simulink model "gen_2_Neel"  (R2017a)
settings: Solver=VariableStepAuto  StartTime=0.0  StopTime=100  MaxStep=1e-4  RelTol=1e-3
libraries: powerlib x33, simrfV2util1 x6, simulink x6, simrfV2_lib x6, powerlib_meascontrol x4
settings Model: SimulationMode=accelerator  Creator=khsva  LastModifiedBy=Purboday Ghosh
settings SolverCC: ZeroCrossAlgorithm=Adaptive
settings OptimizationCC: EfficientMapNaN2IntZero=off
settings HardwareCC: TargetBitPerPointer=64  TargetBitPerSizeT=64  TargetBitPerPtrDiffT=64  TargetLongLongMode=on  TargetIntDivRoundTo=Zero  TargetEndianess=LittleEndian  TargetWordSize=64  TargetHWDeviceType=MATLAB Host  ProdEqTarget=off
settings CodeAppCC: MaxIdLength=128
settings GRTTargetCC: TargetLangStandard=C89/C90 (ANSI)  CombineOutputUpdateFcns=off  GRTInterface=on

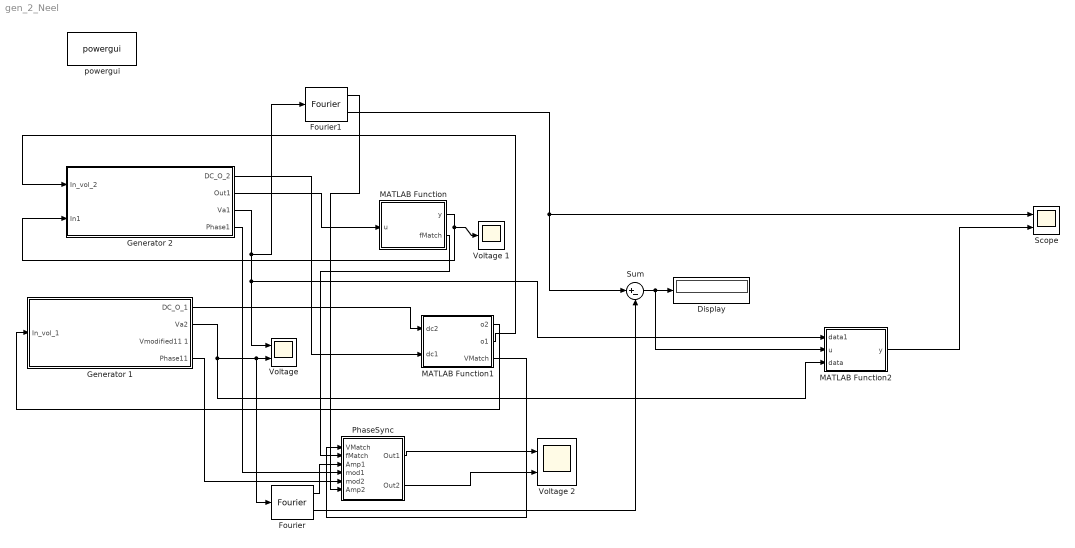
== system gen_2_Neel ==
  Display : Display
  Fourier : powerlib_meascontrol/Measurements/Fourier  Freq=60  n=1  InInit=[0, 0]  Ts=0
      settings: SourceProductName=Simscape Power Systems
  Fourier1 : powerlib_meascontrol/Measurements/Fourier  Freq=60  n=1  InInit=[0, 0]  Ts=0
      settings: SourceProductName=Simscape Power Systems
  "Generator 1 " : Subsystem
  Generator 2 : Subsystem
  MATLAB Function : MATLAB Function  TreatAsAtomicUnit=on
  MATLAB Function1 : MATLAB Function  TreatAsAtomicUnit=on
  MATLAB Function2 : MATLAB Function  TreatAsAtomicUnit=on
  PhaseSync : Subsystem
  Scope : Scope  NumInputPorts=2
  Sum : Sum  Inputs=|+-
  "Voltage " : Scope  NumInputPorts=2
  Voltage 1 : Scope
  Voltage 2 : Scope  NumInputPorts=2
  powergui : powerlib/powergui  Priority=1  SimulationMode=Continuous  SampleTime=50e-6  frequency=60  Iterations=50  frequencyindice=60  Pbase=100e6  ErrMax=1e-4  UnitsV=kV  UnitsW=MW  buscounter=0  FunctionMessages=off  echomessages=off  EnableUseOfTLC=off  CurrentSourceSwitches=off  DisableSnubberDevices=off  DisableRonSwitches=off  DisableVfSwitches=off  DisplayEquations=off  SolverType=Tustin/Backward Euler (TBE)  Interpol=off  ExternalGateDelay=off  methode=off  Ts=100  x0status=blocks  SPID=on  SwTol=0  HookPort=off  RestoreLinks=warning  ResistiveCurrentMeasurement=off  Frange=[0:2:500]  Ylog=off  Xlog=on  ShowGrid=off  save=off  variable=ZData  structure=0  ZoomFFT=off  StartTime=0.0  cycles=1  DisplayStyle=1  fundamental=60  FreqAxis=off  MaxFrequency=1000  frequencyindicesteady=1  RmsSteady=1  display=off
  wires:
  "Generator 1 "/1("DC_O_1 ") -> MATLAB Function1/1(dc2)
  Generator 2/1(DC_O_2) -> MATLAB Function1/2(dc1)
  MATLAB Function1/1(o2) -> "Generator 1 "/1("In_vol_1 ")
  MATLAB Function1/2(o1) -> Generator 2/1("In_vol_2 ")
  MATLAB Function/1(y) -> Voltage 1/1, Generator 2/2(In1)
  Generator 2/2(Out1) -> MATLAB Function/1(u)
  Generator 2/3(Va1) -> Fourier1/1, MATLAB Function2/1(data1), "Voltage "/1
  "Generator 1 "/2("Va2 ") -> MATLAB Function2/3(data), Fourier/1, "Voltage "/2
  Sum/1 -> MATLAB Function2/2(u), Display/1
  Fourier/2 -> Sum/2
  Fourier1/2 -> Sum/1, Scope/1
  MATLAB Function2/1(y) -> Scope/2
  "Generator 1 "/4(Phase11) -> PhaseSync/5(mod2)
  Generator 2/4(Phase1) -> PhaseSync/4(mod1)
  PhaseSync/1(Out1) -> Voltage 2/1
  PhaseSync/2(Out2) -> Voltage 2/2
  Fourier1/1 -> PhaseSync/6(Amp2)
  Fourier/1 -> PhaseSync/3(Amp1)
  MATLAB Function/2(fMatch) -> PhaseSync/2(fMatch)
  MATLAB Function1/3(VMatch) -> PhaseSync/1(VMatch)

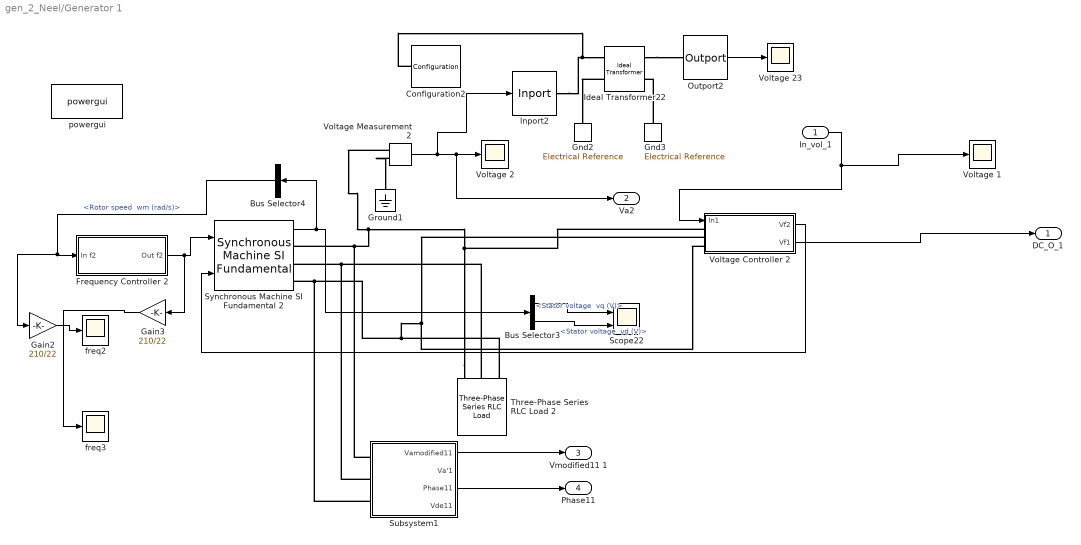
== system gen_2_Neel/Generator 1  ==
  "In_vol_1 " : Inport
  Bus Selector3 : BusSelector  OutputSignals="dq0 components.Stator voltage  vq (V),dq0 components.Stator voltage  vd (V)"
  Bus Selector4 : BusSelector  OutputSignals="Mechanical.Rotor speed  wm (rad/s)"
  Configuration2 : simrfV2util1/Configuration  AutoFreq=on  Tones=[0] Hz  Harmonics=[1]  NormalizeCarrierPower=on  SolverType=Auto  UseCCode=on  StepSize=1e-4 s  AddNoise=on  defaultRNG=on  Seed=0  Temperature=290.0 K  SolverDelFlag=0  AbsTol=1e-6  RelTol=1e-3  MaxIter=10  ErrorEstimationType=2-norm over all variables
      settings: SourceProductName=SimRF  SourceProductBaseCode=RB
  Frequency Controller 2 : Subsystem
  Gain2 : Gain  Gain=210/22
  Gain3 : Gain  Gain=210/22
  Gnd2 : simrfV2_lib/Elements/Electrical Reference
  Gnd3 : simrfV2_lib/Elements/Electrical Reference
  Ground1 : powerlib/Elements/Ground  LConnTagsString=a
  Ideal Transformer22 : simrfV2_lib/Elements/Ideal Transformer  n=10
  Inport2 : simrfV2util1/Inport  SimulinkInputSignalType=Ideal voltage  CarrierFreq=0 Hz  ZS=0  InternalGrounding=on
      settings: SourceProductName=SimRF  SourceProductBaseCode=RB
  Outport2 : simrfV2util1/Outport  SensorType=Ideal voltage  OutputFormat=Complex Baseband  CarrierFreq=0 Hz  ZL=Inf  InternalGrounding=on  StepSize=1e-6 s  AutoStep=on
      settings: SourceProductName=SimRF  SourceProductBaseCode=RB
  Scope22 : Scope  NumInputPorts=2
  Subsystem1 : Subsystem
  Synchronous Machine SI Fundamental 2 : powerlib/Machines/Synchronous Machine SI Fundamental  PresetModel=No  MechanicalLoad=Speed w  ShowDetailedParameters=on  RotorType=Salient-pole  Units=SI fundamental parameters  MeasurementBus=off  NominalParameters="[ 200E3  110   60   70 ]"  Stator="[ 200  3.0892  3.2164  9.7153 ]"  Field="[ 200  30.712 ]"  Dampers2=[ 0.0664, 1.387e-3, 0.0292, 6.896e-4, 7.907e-3, 2.477e-3]  Dampers1="[ 1.1900E-02  4.9076E-04  2.0081E-02  1.0365E-03 ]"  Mechanical=[ 3.895e6 0 20 ]  PolePairs=10  InitialConditions="[ 0  0  0  0  0  0  0  0  0 ]"  SetSaturation=off  Saturation=[695.64,774.7,917.5,1001.6,1082.2,1175.9,1293.6,1430.2,1583.7;9660,10623,12243,13063,13757,14437,15180,15890,16567]  DisplayVfd=off  LoadFlowParameters=[1,0,0,0,0]  TsPowergui=0  TsBlock=-1  IterativeModel=Trapezoidal non iterative  IterativeDiscreteModel=Trapezoidal non iterative  BusType=PV  Pref=0  Qref=0  Qmin=-inf  Qmax=inf  PLF=0  QLF=0
      settings: SourceProductName=Simscape Power Systems  SourceProductBaseCode=PS
  Three-Phase Series RLC Load 2 : powerlib/Elements/Three-Phase Series RLC Load  LConnTagsString=A|B|C  Configuration=Y (grounded)  NominalVoltage=100  Vabc=[1e3 1e3 1e3]  Vabcp=[1e3 1e3 1e3]  NominalFrequency=60  UnbalancedPower=off  ActivePower=2500  InductivePower=0  CapacitivePower=0  Pabc=[10e3 9e3 11e3]  QLabc=[100 90 110]  QCabc=[100 90 110]  Pabcp=[10e3 9e3 11e3]  QLabcp=[100 90 110]  QCabcp=[100 90 110]  Measurements=None  LoadType=constant Z
  Voltage 1 : Scope
  Voltage 2 : Scope
  Voltage 23 : Scope
  Voltage Controller 2 : Subsystem
  Voltage Measurement2 : powerlib/Measurements/Voltage Measurement  PhasorSimulation=off  OutputType=Complex  PSBequivalent=0
  freq2 : Scope
  freq3 : Scope
  powergui : powerlib/powergui  Priority=1  SimulationMode=Continuous  SampleTime=50e-6  frequency=60  Iterations=50  frequencyindice=60  Pbase=100e6  ErrMax=1e-4  UnitsV=kV  UnitsW=MW  buscounter=0  FunctionMessages=off  echomessages=off  EnableUseOfTLC=off  CurrentSourceSwitches=off  DisableSnubberDevices=off  DisableRonSwitches=off  DisableVfSwitches=off  DisplayEquations=off  SolverType=Tustin/Backward Euler (TBE)  Interpol=off  ExternalGateDelay=off  methode=off  Ts=100  x0status=blocks  SPID=on  SwTol=0  HookPort=off  RestoreLinks=warning  ResistiveCurrentMeasurement=off  Frange=[0:2:500]  Ylog=off  Xlog=on  ShowGrid=off  save=off  variable=ZData  structure=0  ZoomFFT=off  StartTime=0.0  cycles=1  DisplayStyle=1  fundamental=60  FreqAxis=off  MaxFrequency=1000  frequencyindicesteady=1  RmsSteady=1  display=off
  "DC_O_1 " : Outport
  "Va2 " : Outport  Port=2
  Vmodified11 1 : Outport  Port=3
  Phase11 : Outport  Port=4
  wires:
  Frequency Controller 2/1(Out f2) -> Gain3/1, Synchronous Machine SI Fundamental 2/1
  Bus Selector3/1 -> Scope22/1  "<Stator voltage  vq (V)>"
  Gain2/1 -> freq2/1
  Synchronous Machine SI Fundamental 2/1 -> Bus Selector4/1, Bus Selector3/1
  Outport2/1 -> Voltage 23/1
  Bus Selector4/1 -> Frequency Controller 2/1(In f2), Gain2/1  "<Rotor speed  wm (rad/s)>"
  Gain3/1 -> freq3/1
  Voltage Measurement2/1 -> Inport2/1, "Va2 "/1, Voltage 2/1
  Voltage Controller 2/1(Vf2) -> Synchronous Machine SI Fundamental 2/2
  Bus Selector3/2 -> Scope22/2  "<Stator voltage  vd (V)>"
  Voltage Controller 2/2(Vf1) -> "DC_O_1 "/1
  "In_vol_1 "/1 -> Voltage 1/1, Voltage Controller 2/1(In1)
  Subsystem1/1(Vamodified11) -> Vmodified11 1/1
  Subsystem1/3(Phase11) -> Phase11/1
  connections:
  Voltage Controller 2/LConn3 -- Voltage Controller 2/LConn2 -- Three-Phase Series RLC Load 2/LConn3 -- Subsystem1/LConn3 -- Synchronous Machine SI Fundamental 2/RConn3
  Voltage Measurement2/LConn2 -- Ground1/LConn1
  Gnd3/LConn1 -- Ideal Transformer22/RConn2
  Inport2/RConn1 -- Configuration2/LConn1 -- Ideal Transformer22/LConn1
  Three-Phase Series RLC Load 2/LConn2 -- Subsystem1/LConn2 -- Synchronous Machine SI Fundamental 2/RConn2
  Ideal Transformer22/RConn1 -- Outport2/LConn1
  Three-Phase Series RLC Load 2/LConn1 -- Voltage Controller 2/LConn1 -- Subsystem1/LConn1 -- Synchronous Machine SI Fundamental 2/RConn1 -- Voltage Measurement2/LConn1
  Ideal Transformer22/LConn2 -- Gnd2/LConn1

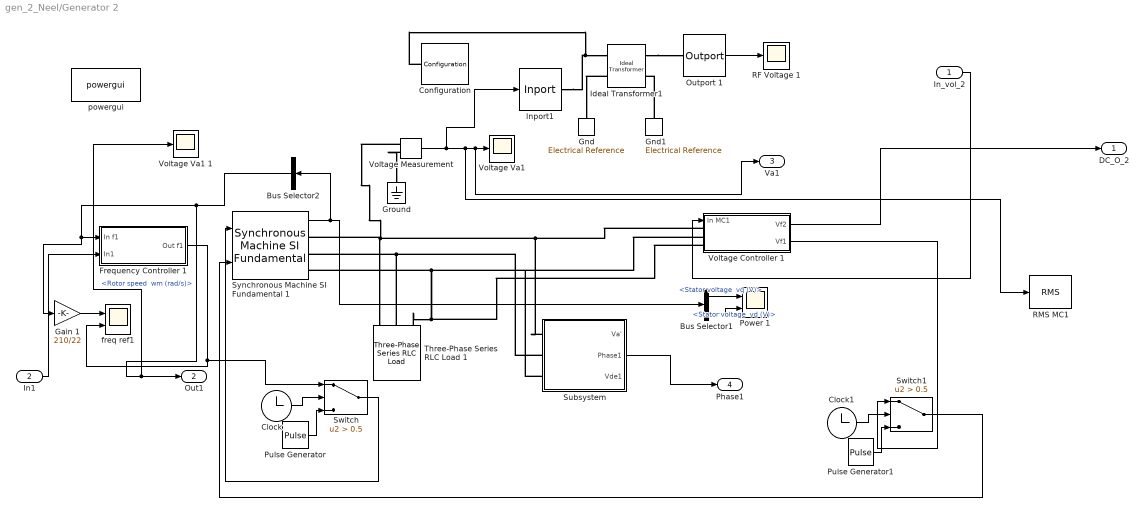
== system gen_2_Neel/Generator 2 ==
  "In_vol_2 " : Inport
  In1 : Inport  Port=2
  Bus Selector1 : BusSelector  OutputSignals="dq0 components.Stator voltage  vq (V),dq0 components.Stator voltage  vd (V)"
  Bus Selector2 : BusSelector  OutputSignals="Mechanical.Rotor speed  wm (rad/s)"
  Clock : Clock
  Clock1 : Clock
  Configuration : simrfV2util1/Configuration  AutoFreq=on  Tones=[0] Hz  Harmonics=[1]  NormalizeCarrierPower=on  SolverType=Auto  UseCCode=on  StepSize=1e-4 s  AddNoise=on  defaultRNG=on  Seed=0  Temperature=290.0 K  SolverDelFlag=0  AbsTol=1e-6  RelTol=1e-3  MaxIter=10  ErrorEstimationType=2-norm over all variables
      settings: SourceProductName=SimRF  SourceProductBaseCode=RB
  Frequency Controller 1 : Subsystem
  Gain 1 : Gain  Gain=210/22
  Gnd : simrfV2_lib/Elements/Electrical Reference
  Gnd1 : simrfV2_lib/Elements/Electrical Reference
  Ground : powerlib/Elements/Ground  LConnTagsString=a
  Ideal Transformer1 : simrfV2_lib/Elements/Ideal Transformer  n=10
  Inport1 : simrfV2util1/Inport  SimulinkInputSignalType=Ideal voltage  CarrierFreq=0 Hz  ZS=0  InternalGrounding=on
      settings: SourceProductName=SimRF  SourceProductBaseCode=RB
  Outport 1 : simrfV2util1/Outport  SensorType=Ideal voltage  OutputFormat=Complex Baseband  CarrierFreq=0 Hz  ZL=Inf  InternalGrounding=on  StepSize=1e-6 s  AutoStep=on
      settings: SourceProductName=SimRF  SourceProductBaseCode=RB
  Power 1 : Scope  NumInputPorts=2
  Pulse Generator : DiscretePulseGenerator  PulseType=Time based  Amplitude=0  Period=5  PulseWidth=99.99  PhaseDelay=0.5
  Pulse Generator1 : DiscretePulseGenerator  PulseType=Time based  Amplitude=0  Period=5  PulseWidth=99.99  PhaseDelay=0.5
  RF Voltage 1 : Scope
  RMS MC1 : powerlib_meascontrol/Measurements/RMS  TrueRMS=on  Freq=60  RMSInit=120  Ts=0
  Subsystem : Subsystem
  Switch : Switch  Criteria=u2 > Threshold  Threshold=0.5
  Switch1 : Switch  Criteria=u2 > Threshold  Threshold=0.5
  Synchronous Machine SI Fundamental 1 : powerlib/Machines/Synchronous Machine SI Fundamental  PresetModel=No  MechanicalLoad=Speed w  ShowDetailedParameters=on  RotorType=Salient-pole  Units=SI fundamental parameters  MeasurementBus=off  NominalParameters="[ 200E3  110   60   70 ]"  Stator="[ 200  3.0892  3.2164  9.7153 ]"  Field="[ 200  30.712 ]"  Dampers2=[ 0.0664, 1.387e-3, 0.0292, 6.896e-4, 7.907e-3, 2.477e-3]  Dampers1="[ 1.1900E-02  4.9076E-04  2.0081E-02  1.0365E-03 ]"  Mechanical=[ 3.895e6 0 20 ]  PolePairs=10  InitialConditions="[ 0  0  0  0  0  0  0  0  0 ]"  SetSaturation=off  Saturation=[695.64,774.7,917.5,1001.6,1082.2,1175.9,1293.6,1430.2,1583.7;9660,10623,12243,13063,13757,14437,15180,15890,16567]  DisplayVfd=off  LoadFlowParameters=[1,0,0,0,0]  TsPowergui=0  TsBlock=-1  IterativeModel=Trapezoidal non iterative  IterativeDiscreteModel=Trapezoidal non iterative  BusType=PV  Pref=0  Qref=0  Qmin=-inf  Qmax=inf  PLF=0  QLF=0
      settings: SourceProductName=Simscape Power Systems  SourceProductBaseCode=PS
  Three-Phase Series RLC Load 1 : powerlib/Elements/Three-Phase Series RLC Load  LConnTagsString=A|B|C  Configuration=Y (grounded)  NominalVoltage=100  Vabc=[1e3 1e3 1e3]  Vabcp=[1e3 1e3 1e3]  NominalFrequency=60  UnbalancedPower=off  ActivePower=1000  InductivePower=0  CapacitivePower=0  Pabc=[10e3 9e3 11e3]  QLabc=[100 90 110]  QCabc=[100 90 110]  Pabcp=[10e3 9e3 11e3]  QLabcp=[100 90 110]  QCabcp=[100 90 110]  Measurements=None  LoadType=constant Z
  Voltage Controller 1 : Subsystem
  Voltage Measurement : powerlib/Measurements/Voltage Measurement  PhasorSimulation=off  OutputType=Complex  PSBequivalent=0
  "Voltage Va1 " : Scope
  Voltage Va1 1 : Scope
  "freq ref1 " : Scope  NumInputPorts=2
  powergui : powerlib/powergui  Priority=1  SimulationMode=Continuous  SampleTime=50e-6  frequency=60  Iterations=50  frequencyindice=60  Pbase=100e6  ErrMax=1e-4  UnitsV=kV  UnitsW=MW  buscounter=0  FunctionMessages=off  echomessages=off  EnableUseOfTLC=off  CurrentSourceSwitches=off  DisableSnubberDevices=off  DisableRonSwitches=off  DisableVfSwitches=off  DisplayEquations=off  SolverType=Tustin/Backward Euler (TBE)  Interpol=off  ExternalGateDelay=off  methode=off  Ts=100  x0status=blocks  SPID=on  SwTol=0  HookPort=off  RestoreLinks=warning  ResistiveCurrentMeasurement=off  Frange=[0:2:500]  Ylog=off  Xlog=on  ShowGrid=off  save=off  variable=ZData  structure=0  ZoomFFT=off  StartTime=0.0  cycles=1  DisplayStyle=1  fundamental=60  FreqAxis=off  MaxFrequency=1000  frequencyindicesteady=1  RmsSteady=1  display=off
  DC_O_2 : Outport
  Out1 : Outport  Port=2
  Va1 : Outport  Port=3
  Phase1 : Outport  Port=4
  wires:
  Outport 1/1 -> RF Voltage 1/1
  Synchronous Machine SI Fundamental 1/1 -> Bus Selector2/1, Bus Selector1/1
  Gain 1/1 -> "freq ref1 "/1
  Frequency Controller 1/1(Out f1) -> Switch/1, "freq ref1 "/2
  Bus Selector1/1 -> Power 1/1  "<Stator voltage  vq (V)>"
  Bus Selector1/2 -> Power 1/2  "<Stator voltage  vd (V)>"
  Bus Selector2/1 -> Voltage Va1 1/1, Out1/1, Gain 1/1, Frequency Controller 1/1(In f1)  "<Rotor speed  wm (rad/s)>"
  "In_vol_2 "/1 -> Voltage Controller 1/1(In MC1)
  Voltage Measurement/1 -> Inport1/1, RMS MC1/1, Va1/1, "Voltage Va1 "/1
  Voltage Controller 1/1(Vf2) -> DC_O_2/1
  In1/1 -> Frequency Controller 1/2(In1)
  Clock/1 -> Switch/2
  Switch/1 -> Synchronous Machine SI Fundamental 1/1
  Pulse Generator/1 -> Switch/3
  Pulse Generator1/1 -> Switch1/3
  Clock1/1 -> Switch1/2
  Switch1/1 -> Synchronous Machine SI Fundamental 1/2
  Voltage Controller 1/2(Vf1) -> Switch1/1
  Subsystem/2(Phase1) -> Phase1/1
  connections:
  Inport1/RConn1 -- Configuration/LConn1 -- Ideal Transformer1/LConn1
  Ideal Transformer1/RConn1 -- Outport 1/LConn1
  Ideal Transformer1/LConn2 -- Gnd/LConn1
  Gnd1/LConn1 -- Ideal Transformer1/RConn2
  Voltage Controller 1/LConn1 -- Subsystem/LConn1 -- Voltage Measurement/LConn1 -- Synchronous Machine SI Fundamental 1/RConn1 -- Three-Phase Series RLC Load 1/LConn1
  Voltage Measurement/LConn2 -- Ground/LConn1
  Three-Phase Series RLC Load 1/LConn3 -- Subsystem/LConn3 -- Voltage Controller 1/LConn2 -- Synchronous Machine SI Fundamental 1/RConn3 -- Voltage Controller 1/LConn3
  Three-Phase Series RLC Load 1/LConn2 -- Synchronous Machine SI Fundamental 1/RConn2 -- Subsystem/LConn2

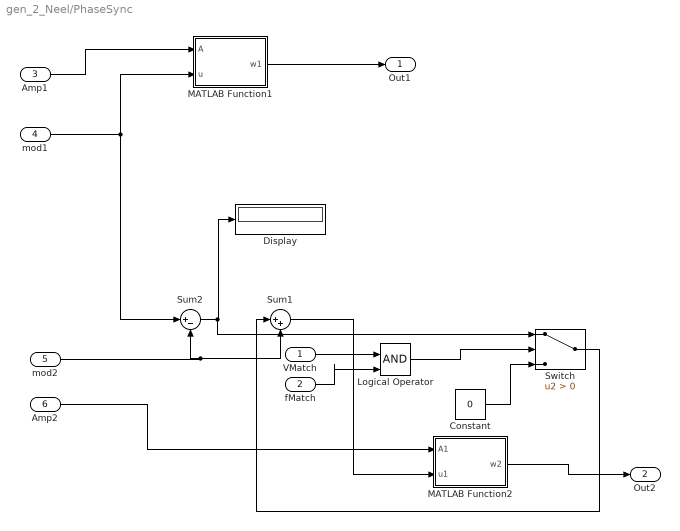
== system gen_2_Neel/PhaseSync ==
  VMatch : Inport
  fMatch : Inport  Port=2
  Amp1 : Inport  Port=3
  mod1 : Inport  Port=4
  mod2 : Inport  Port=5
  Amp2 : Inport  Port=6
  Constant : Constant  Value=0
  Display : Display
  Logical Operator : Logic  IconShape=distinctive  AllPortsSameDT=off  OutDataTypeStr=boolean
  MATLAB Function1 : MATLAB Function  TreatAsAtomicUnit=on
  MATLAB Function2 : MATLAB Function  TreatAsAtomicUnit=on
  Sum1 : Sum  Inputs=|++
  Sum2 : Sum  Inputs=|+-
  Switch : Switch  Criteria=u2 > Threshold
  Out1 : Outport
  Out2 : Outport  Port=2
  wires:
  Sum2/1 -> Switch/1, Display/1
  Sum1/1 -> MATLAB Function2/2(u1)
  MATLAB Function2/1(w2) -> Out2/1
  MATLAB Function1/1(w1) -> Out1/1
  Amp1/1 -> MATLAB Function1/1(A)
  Amp2/1 -> MATLAB Function2/1(A1)
  mod2/1 -> Sum1/2, Sum2/2
  Logical Operator/1 -> Switch/2
  Constant/1 -> Switch/3
  Switch/1 -> Sum1/1
  mod1/1 -> MATLAB Function1/2(u), Sum2/1
  fMatch/1 -> Logical Operator/2
  VMatch/1 -> Logical Operator/1

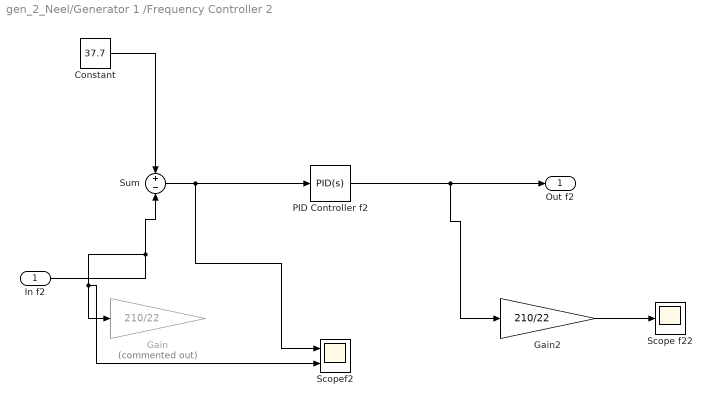
== system gen_2_Neel/Generator 1 /Frequency Controller 2 ==
  In f2 : Inport
  Constant : Constant  Value=37.7
  Gain : Gain  Commented=on  Gain=210/22
  Gain2 : Gain  Gain=210/22
  PID Controller f2 : simulink/Continuous/PID Controller  Controller=PID  TimeDomain=Continuous-time  SampleTime=-1  IntegratorMethod=Forward Euler  FilterMethod=Forward Euler  Form=Ideal  UseFilter=on  ControllerParametersSource=internal  P=9.99999998333334e-05  I=6309.57342377002  D=0  N=100  InitialConditionSource=internal  InitialConditionForIntegrator=0  InitialConditionForFilter=0  ExternalReset=none  LimitOutput=off  UpperSaturationLimit=inf  LowerSaturationLimit=-inf  LinearizeAsGain=on  AntiWindupMode=none  Kb=1  TrackingMode=off  Kt=1  PParamMin=[]  PParamMax=[]  IParamMin=[]  IParamMax=[]  DParamMin=[]  DParamMax=[]  NParamMin=[]  NParamMax=[]  KbParamMin=[]  KbParamMax=[]  KtParamMin=[]  KtParamMax=[]  POutMin=[]  POutMax=[]  IOutMin=[]  IOutMax=[]  DOutMin=[]  DOutMax=[]  NOutMin=[]  NOutMax=[]  KbOutMin=[]  KbOutMax=[]  KtOutMin=[]  KtOutMax=[]  IntegratorOutMin=[]  IntegratorOutMax=[]  FilterOutMin=[]  FilterOutMax=[]  SumOutMin=[]  SumOutMax=[]  SumI1OutMin=[]  SumI1OutMax=[]  SumI2OutMin=[]  SumI2OutMax=[]  SumI3OutMin=[]  SumI3OutMax=[]  SumDOutMin=[]  SumDOutMax=[]  SaturationOutMin=[]  SaturationOutMax=[]  IntegratorContinuousStateAttributes=''  IntegratorStateMustResolveToSignalObject=off  IntegratorRTWStateStorageClass=Auto  FilterContinuousStateAttributes=''  FilterStateMustResolveToSignalObject=off  FilterRTWStateStorageClass=Auto  DifferentiatorICPrevScaledInput=0  DifferentiatorOutMin=[]  DifferentiatorOutMax=[]  InitialConditionSetting=State (most efficient)
  Scope f22 : Scope
  Scopef2 : Scope  NumInputPorts=2
  Sum : Sum  Inputs=+-
  Out f2 : Outport
  wires:
  In f2/1 -> Sum/2, Scopef2/2, Gain/1
  Sum/1 -> PID Controller f2/1, Scopef2/1
  PID Controller f2/1 -> Gain2/1, Out f2/1
  Gain2/1 -> Scope f22/1
  Constant/1 -> Sum/1

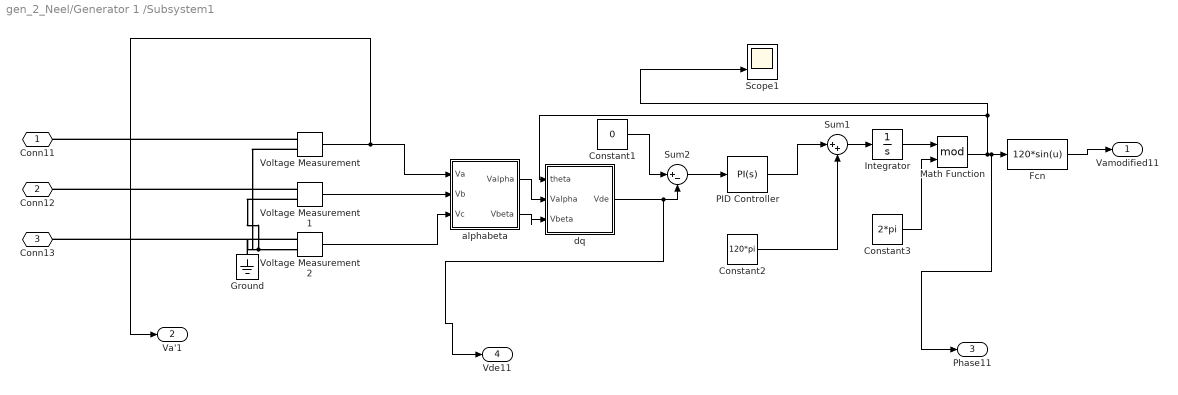
== system gen_2_Neel/Generator 1 /Subsystem1 ==
  Constant1 : Constant  Value=0
  Constant2 : Constant  Value=120*pi
  Constant3 : Constant  Value=2*pi
  Fcn : Fcn  Expr=120*sin(u)
  Ground : powerlib/Elements/Ground  LConnTagsString=a
  Integrator : Integrator
  Math Function : Math  Operator=mod  SaturateOnIntegerOverflow=on
  PID Controller : simulink/Continuous/PID Controller  Controller=PI  TimeDomain=Continuous-time  SampleTime=-1  IntegratorMethod=Forward Euler  FilterMethod=Forward Euler  Form=Parallel  UseFilter=on  ControllerParametersSource=internal  P=1  I=1  D=0  N=100  InitialConditionSource=internal  InitialConditionForIntegrator=0  InitialConditionForFilter=0  ExternalReset=none  LimitOutput=off  UpperSaturationLimit=inf  LowerSaturationLimit=-inf  LinearizeAsGain=on  AntiWindupMode=none  Kb=1  TrackingMode=off  Kt=1  PParamMin=[]  PParamMax=[]  IParamMin=[]  IParamMax=[]  DParamMin=[]  DParamMax=[]  NParamMin=[]  NParamMax=[]  KbParamMin=[]  KbParamMax=[]  KtParamMin=[]  KtParamMax=[]  POutMin=[]  POutMax=[]  IOutMin=[]  IOutMax=[]  DOutMin=[]  DOutMax=[]  NOutMin=[]  NOutMax=[]  KbOutMin=[]  KbOutMax=[]  KtOutMin=[]  KtOutMax=[]  IntegratorOutMin=[]  IntegratorOutMax=[]  FilterOutMin=[]  FilterOutMax=[]  SumOutMin=[]  SumOutMax=[]  SumI1OutMin=[]  SumI1OutMax=[]  SumI2OutMin=[]  SumI2OutMax=[]  SumI3OutMin=[]  SumI3OutMax=[]  SumDOutMin=[]  SumDOutMax=[]  SaturationOutMin=[]  SaturationOutMax=[]  IntegratorContinuousStateAttributes=''  IntegratorStateMustResolveToSignalObject=off  IntegratorRTWStateStorageClass=Auto  FilterContinuousStateAttributes=''  FilterStateMustResolveToSignalObject=off  FilterRTWStateStorageClass=Auto  DifferentiatorICPrevScaledInput=0  DifferentiatorOutMin=[]  DifferentiatorOutMax=[]  InitialConditionSetting=State (most efficient)
  Scope1 : Scope  NumInputPorts=2
  Sum1 : Sum  Inputs=|++
  Sum2 : Sum  Inputs=|+-
  Voltage Measurement : powerlib/Measurements/Voltage Measurement  PhasorSimulation=off  OutputType=Complex  PSBequivalent=0
  Voltage Measurement1 : powerlib/Measurements/Voltage Measurement  PhasorSimulation=off  OutputType=Complex  PSBequivalent=0
  Voltage Measurement2 : powerlib/Measurements/Voltage Measurement  PhasorSimulation=off  OutputType=Complex  PSBequivalent=0
  alphabeta : Subsystem
  dq : Subsystem
  Conn11 : PMIOPort  Port=1  Side=Left
  Conn12 : PMIOPort  Port=2  Side=Left
  Conn13 : PMIOPort  Port=3  Side=Left
  Vamodified11 : Outport
  Va'1 : Outport  Port=2
  Phase11 : Outport  Port=3
  Vde11 : Outport  Port=4
  wires:
  Sum2/1 -> PID Controller/1
  Voltage Measurement2/1 -> alphabeta/3(Vc)
  Constant3/1 -> Math Function/2
  Integrator/1 -> Math Function/1
  Math Function/1 -> dq/1(theta), Scope1/2, Phase11/1, Fcn/1
  Fcn/1 -> Vamodified11/1
  Sum1/1 -> Integrator/1
  Voltage Measurement1/1 -> alphabeta/2(Vb)
  alphabeta/1(Valpha) -> dq/2(Valpha)
  Voltage Measurement/1 -> Va'1/1, alphabeta/1(Va)
  Constant2/1 -> Sum1/2
  alphabeta/2(Vbeta) -> dq/3(Vbeta)
  dq/1(Vde) -> Vde11/1, Sum2/2
  PID Controller/1 -> Sum1/1
  Constant1/1 -> Sum2/1
  connections:
  Voltage Measurement1/LConn1 -- Conn12/RConn1
  Voltage Measurement/LConn1 -- Conn11/RConn1
  Voltage Measurement2/LConn1 -- Conn13/RConn1
  Ground/LConn1 -- Voltage Measurement/LConn2 -- Voltage Measurement1/LConn2 -- Voltage Measurement2/LConn2

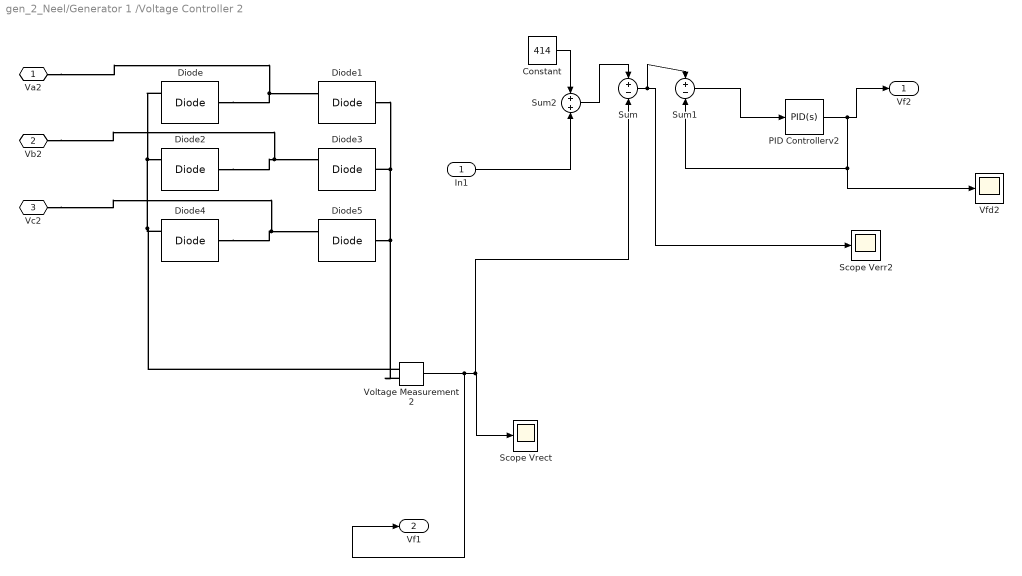
== system gen_2_Neel/Generator 1 /Voltage Controller 2 ==
  In1 : Inport
  Constant : Constant  Value=414
  Diode{,1..5} (6 alike) : powerlib/Power Electronics/Diode  Ron=0.001  Lon=0  Vf=0.8  IC=0  UseSnubber=0  Rs=500  Cs=250e-9  Measurements=on
  PID Controllerv2 : simulink/Continuous/PID Controller  Controller=PID  TimeDomain=Continuous-time  SampleTime=-1  IntegratorMethod=Forward Euler  FilterMethod=Forward Euler  Form=Parallel  UseFilter=on  ControllerParametersSource=internal  P=0  I=1.00000000010753  D=0  N=100  InitialConditionSource=internal  InitialConditionForIntegrator=0  InitialConditionForFilter=0  ExternalReset=none  LimitOutput=off  UpperSaturationLimit=inf  LowerSaturationLimit=-inf  LinearizeAsGain=on  AntiWindupMode=none  Kb=1  TrackingMode=off  Kt=1  PParamMin=[]  PParamMax=[]  IParamMin=[]  IParamMax=[]  DParamMin=[]  DParamMax=[]  NParamMin=[]  NParamMax=[]  KbParamMin=[]  KbParamMax=[]  KtParamMin=[]  KtParamMax=[]  POutMin=[]  POutMax=[]  IOutMin=[]  IOutMax=[]  DOutMin=[]  DOutMax=[]  NOutMin=[]  NOutMax=[]  KbOutMin=[]  KbOutMax=[]  KtOutMin=[]  KtOutMax=[]  IntegratorOutMin=[]  IntegratorOutMax=[]  FilterOutMin=[]  FilterOutMax=[]  SumOutMin=[]  SumOutMax=[]  SumI1OutMin=[]  SumI1OutMax=[]  SumI2OutMin=[]  SumI2OutMax=[]  SumI3OutMin=[]  SumI3OutMax=[]  SumDOutMin=[]  SumDOutMax=[]  SaturationOutMin=[]  SaturationOutMax=[]  IntegratorContinuousStateAttributes=''  IntegratorStateMustResolveToSignalObject=off  IntegratorRTWStateStorageClass=Auto  FilterContinuousStateAttributes=''  FilterStateMustResolveToSignalObject=off  FilterRTWStateStorageClass=Auto  DifferentiatorICPrevScaledInput=0  DifferentiatorOutMin=[]  DifferentiatorOutMax=[]  InitialConditionSetting=State (most efficient)
  Scope Verr2 : Scope
  Scope Vrect : Scope
  Sum : Sum  Inputs=+-
  Sum1 : Sum  Inputs=+-
  Sum2 : Sum
  Vfd2 : Scope
  Voltage Measurement2 : powerlib/Measurements/Voltage Measurement  PhasorSimulation=off  OutputType=Complex  PSBequivalent=0
  Va2 : PMIOPort  Port=1  Side=Left
  Vb2 : PMIOPort  Port=2  Side=Left
  Vc2 : PMIOPort  Port=3  Side=Left
  Vf2 : Outport
  Vf1 : Outport  Port=2
  wires:
  Constant/1 -> Sum2/1
  Voltage Measurement2/1 -> Vf1/1, Sum/2, Scope Vrect/1
  PID Controllerv2/1 -> Sum1/2, Vfd2/1, Vf2/1
  Sum/1 -> Sum1/1, Scope Verr2/1
  Sum1/1 -> PID Controllerv2/1
  Sum2/1 -> Sum/1
  In1/1 -> Sum2/2
  connections:
  Diode1/LConn1 -- Voltage Measurement2/LConn2 -- Diode5/LConn1 -- Diode3/LConn1
  Diode/LConn1 -- Va2/RConn1 -- Diode1/RConn1
  Diode2/LConn1 -- Vb2/RConn1 -- Diode3/RConn1
  Diode4/LConn1 -- Vc2/RConn1 -- Diode5/RConn1
  Diode/RConn1 -- Voltage Measurement2/LConn1 -- Diode4/RConn1 -- Diode2/RConn1

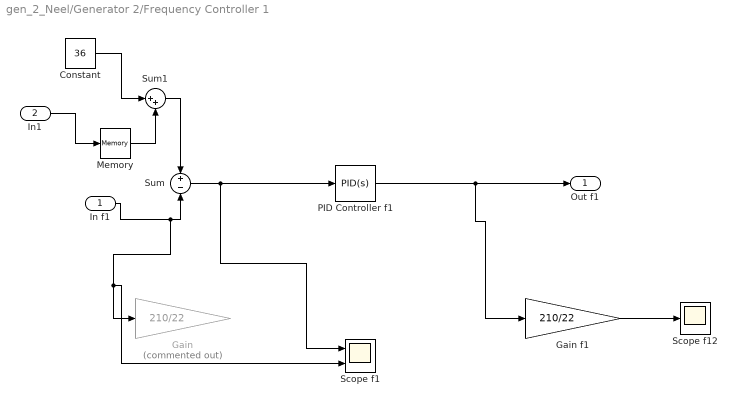
== system gen_2_Neel/Generator 2/Frequency Controller 1 ==
  In f1 : Inport
  In1 : Inport  Port=2
  Constant : Constant  Value=36
  Gain : Gain  Commented=on  Gain=210/22
  Gain f1 : Gain  Gain=210/22
  Memory : Memory
  PID Controller f1 : simulink/Continuous/PID Controller  Controller=PID  TimeDomain=Continuous-time  SampleTime=-1  IntegratorMethod=Forward Euler  FilterMethod=Forward Euler  Form=Ideal  UseFilter=on  ControllerParametersSource=internal  P=9.99999998333334e-05  I=6309.57342377002  D=0  N=100  InitialConditionSource=internal  InitialConditionForIntegrator=0  InitialConditionForFilter=0  ExternalReset=none  LimitOutput=off  UpperSaturationLimit=inf  LowerSaturationLimit=-inf  LinearizeAsGain=on  AntiWindupMode=none  Kb=1  TrackingMode=off  Kt=1  PParamMin=[]  PParamMax=[]  IParamMin=[]  IParamMax=[]  DParamMin=[]  DParamMax=[]  NParamMin=[]  NParamMax=[]  KbParamMin=[]  KbParamMax=[]  KtParamMin=[]  KtParamMax=[]  POutMin=[]  POutMax=[]  IOutMin=[]  IOutMax=[]  DOutMin=[]  DOutMax=[]  NOutMin=[]  NOutMax=[]  KbOutMin=[]  KbOutMax=[]  KtOutMin=[]  KtOutMax=[]  IntegratorOutMin=[]  IntegratorOutMax=[]  FilterOutMin=[]  FilterOutMax=[]  SumOutMin=[]  SumOutMax=[]  SumI1OutMin=[]  SumI1OutMax=[]  SumI2OutMin=[]  SumI2OutMax=[]  SumI3OutMin=[]  SumI3OutMax=[]  SumDOutMin=[]  SumDOutMax=[]  SaturationOutMin=[]  SaturationOutMax=[]  IntegratorContinuousStateAttributes=''  IntegratorStateMustResolveToSignalObject=off  IntegratorRTWStateStorageClass=Auto  FilterContinuousStateAttributes=''  FilterStateMustResolveToSignalObject=off  FilterRTWStateStorageClass=Auto  DifferentiatorICPrevScaledInput=0  DifferentiatorOutMin=[]  DifferentiatorOutMax=[]  InitialConditionSetting=State (most efficient)
  Scope f1 : Scope  NumInputPorts=2
  Scope f12 : Scope
  Sum : Sum  Inputs=+-
  Sum1 : Sum  Inputs=|++
  Out f1 : Outport
  wires:
  In f1/1 -> Scope f1/2, Gain/1, Sum/2
  Sum/1 -> PID Controller f1/1, Scope f1/1
  PID Controller f1/1 -> Gain f1/1, Out f1/1
  Gain f1/1 -> Scope f12/1
  Constant/1 -> Sum1/1
  Sum1/1 -> Sum/1
  Memory/1 -> Sum1/2
  In1/1 -> Memory/1

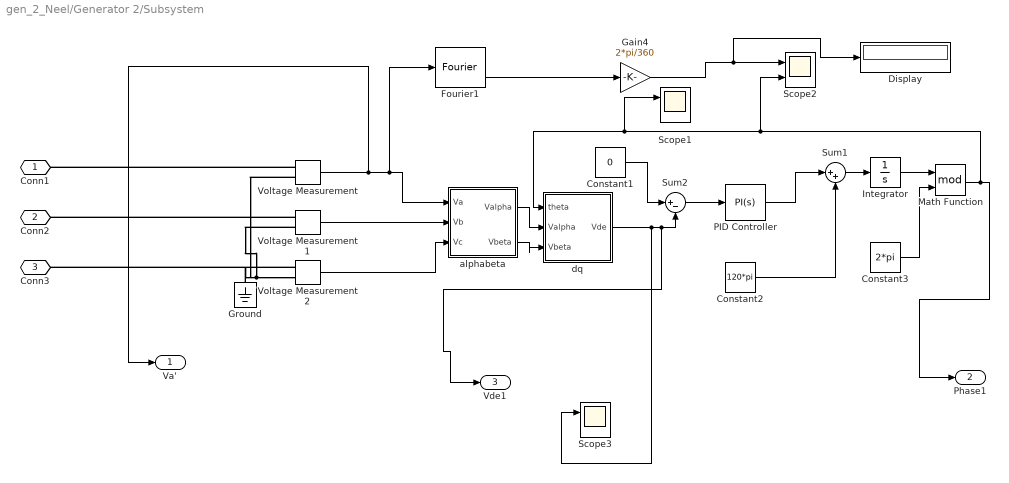
== system gen_2_Neel/Generator 2/Subsystem ==
  Constant1 : Constant  Value=0
  Constant2 : Constant  Value=120*pi
  Constant3 : Constant  Value=2*pi
  Display : Display
  Fourier1 : powerlib_meascontrol/Measurements/Fourier  Freq=60  n=1  InInit=[0, 0]  Ts=0
      settings: SourceProductName=Simscape Power Systems
  Gain4 : Gain  Gain=2*pi/360
  Ground : powerlib/Elements/Ground  LConnTagsString=a
  Integrator : Integrator
  Math Function : Math  Operator=mod  SaturateOnIntegerOverflow=on
  PID Controller : simulink/Continuous/PID Controller  Controller=PI  TimeDomain=Continuous-time  SampleTime=-1  IntegratorMethod=Forward Euler  FilterMethod=Forward Euler  Form=Parallel  UseFilter=on  ControllerParametersSource=internal  P=1  I=1  D=0  N=100  InitialConditionSource=internal  InitialConditionForIntegrator=0  InitialConditionForFilter=0  ExternalReset=none  LimitOutput=off  UpperSaturationLimit=inf  LowerSaturationLimit=-inf  LinearizeAsGain=on  AntiWindupMode=none  Kb=1  TrackingMode=off  Kt=1  PParamMin=[]  PParamMax=[]  IParamMin=[]  IParamMax=[]  DParamMin=[]  DParamMax=[]  NParamMin=[]  NParamMax=[]  KbParamMin=[]  KbParamMax=[]  KtParamMin=[]  KtParamMax=[]  POutMin=[]  POutMax=[]  IOutMin=[]  IOutMax=[]  DOutMin=[]  DOutMax=[]  NOutMin=[]  NOutMax=[]  KbOutMin=[]  KbOutMax=[]  KtOutMin=[]  KtOutMax=[]  IntegratorOutMin=[]  IntegratorOutMax=[]  FilterOutMin=[]  FilterOutMax=[]  SumOutMin=[]  SumOutMax=[]  SumI1OutMin=[]  SumI1OutMax=[]  SumI2OutMin=[]  SumI2OutMax=[]  SumI3OutMin=[]  SumI3OutMax=[]  SumDOutMin=[]  SumDOutMax=[]  SaturationOutMin=[]  SaturationOutMax=[]  IntegratorContinuousStateAttributes=''  IntegratorStateMustResolveToSignalObject=off  IntegratorRTWStateStorageClass=Auto  FilterContinuousStateAttributes=''  FilterStateMustResolveToSignalObject=off  FilterRTWStateStorageClass=Auto  DifferentiatorICPrevScaledInput=0  DifferentiatorOutMin=[]  DifferentiatorOutMax=[]  InitialConditionSetting=State (most efficient)
  Scope1 : Scope  NumInputPorts=2
  Scope2 : Scope  NumInputPorts=2
  Scope3 : Scope  NumInputPorts=2
  Sum1 : Sum  Inputs=|++
  Sum2 : Sum  Inputs=|+-
  Voltage Measurement : powerlib/Measurements/Voltage Measurement  PhasorSimulation=off  OutputType=Complex  PSBequivalent=0
  Voltage Measurement1 : powerlib/Measurements/Voltage Measurement  PhasorSimulation=off  OutputType=Complex  PSBequivalent=0
  Voltage Measurement2 : powerlib/Measurements/Voltage Measurement  PhasorSimulation=off  OutputType=Complex  PSBequivalent=0
  alphabeta : Subsystem
  dq : Subsystem
  Conn1 : PMIOPort  Port=1  Side=Left
  Conn2 : PMIOPort  Port=2  Side=Left
  Conn3 : PMIOPort  Port=3  Side=Left
  Va' : Outport
  Phase1 : Outport  Port=2
  Vde1 : Outport  Port=3
  wires:
  Sum2/1 -> PID Controller/1
  Voltage Measurement2/1 -> alphabeta/3(Vc)
  Constant3/1 -> Math Function/2
  Integrator/1 -> Math Function/1
  Math Function/1 -> Phase1/1, Scope2/2, Scope1/1, dq/1(theta)
  Sum1/1 -> Integrator/1
  Voltage Measurement1/1 -> alphabeta/2(Vb)
  alphabeta/1(Valpha) -> dq/2(Valpha)
  Voltage Measurement/1 -> Va'/1, Fourier1/1, alphabeta/1(Va)
  Constant2/1 -> Sum1/2
  alphabeta/2(Vbeta) -> dq/3(Vbeta)
  dq/1(Vde) -> Scope3/1, Vde1/1, Sum2/2
  PID Controller/1 -> Sum1/1
  Constant1/1 -> Sum2/1
  Fourier1/2 -> Gain4/1
  Gain4/1 -> Display/1, Scope2/1
  connections:
  Voltage Measurement1/LConn1 -- Conn2/RConn1
  Voltage Measurement/LConn1 -- Conn1/RConn1
  Voltage Measurement2/LConn1 -- Conn3/RConn1
  Ground/LConn1 -- Voltage Measurement/LConn2 -- Voltage Measurement1/LConn2 -- Voltage Measurement2/LConn2

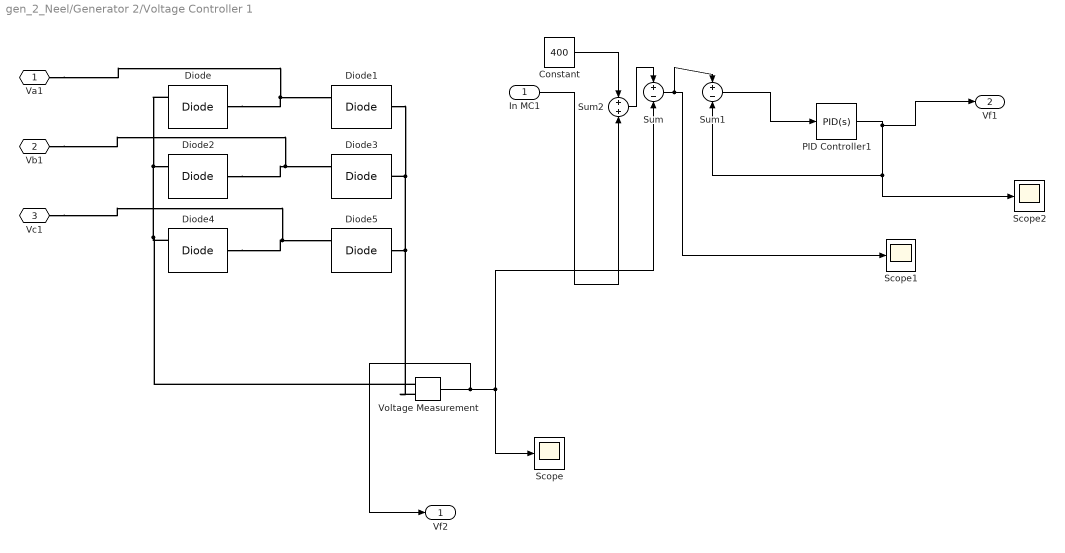
== system gen_2_Neel/Generator 2/Voltage Controller 1 ==
  In MC1 : Inport
  Constant : Constant  Value=400
  Diode{,1..5} (6 alike) : powerlib/Power Electronics/Diode  Ron=0.001  Lon=0  Vf=0.8  IC=0  UseSnubber=0  Rs=500  Cs=250e-9  Measurements=on
  PID Controller1 : simulink/Continuous/PID Controller  Controller=PID  TimeDomain=Continuous-time  SampleTime=-1  IntegratorMethod=Forward Euler  FilterMethod=Forward Euler  Form=Parallel  UseFilter=on  ControllerParametersSource=internal  P=0  I=1.00000000010753  D=0  N=100  InitialConditionSource=internal  InitialConditionForIntegrator=0  InitialConditionForFilter=0  ExternalReset=none  LimitOutput=off  UpperSaturationLimit=inf  LowerSaturationLimit=-inf  LinearizeAsGain=on  AntiWindupMode=none  Kb=1  TrackingMode=off  Kt=1  PParamMin=[]  PParamMax=[]  IParamMin=[]  IParamMax=[]  DParamMin=[]  DParamMax=[]  NParamMin=[]  NParamMax=[]  KbParamMin=[]  KbParamMax=[]  KtParamMin=[]  KtParamMax=[]  POutMin=[]  POutMax=[]  IOutMin=[]  IOutMax=[]  DOutMin=[]  DOutMax=[]  NOutMin=[]  NOutMax=[]  KbOutMin=[]  KbOutMax=[]  KtOutMin=[]  KtOutMax=[]  IntegratorOutMin=[]  IntegratorOutMax=[]  FilterOutMin=[]  FilterOutMax=[]  SumOutMin=[]  SumOutMax=[]  SumI1OutMin=[]  SumI1OutMax=[]  SumI2OutMin=[]  SumI2OutMax=[]  SumI3OutMin=[]  SumI3OutMax=[]  SumDOutMin=[]  SumDOutMax=[]  SaturationOutMin=[]  SaturationOutMax=[]  IntegratorContinuousStateAttributes=''  IntegratorStateMustResolveToSignalObject=off  IntegratorRTWStateStorageClass=Auto  FilterContinuousStateAttributes=''  FilterStateMustResolveToSignalObject=off  FilterRTWStateStorageClass=Auto  DifferentiatorICPrevScaledInput=0  DifferentiatorOutMin=[]  DifferentiatorOutMax=[]  InitialConditionSetting=State (most efficient)
  Scope : Scope
  Scope1 : Scope
  Scope2 : Scope
  Sum : Sum  Inputs=+-
  Sum1 : Sum  Inputs=+-
  Sum2 : Sum
  Voltage Measurement : powerlib/Measurements/Voltage Measurement  PhasorSimulation=off  OutputType=Complex  PSBequivalent=0
  Va1 : PMIOPort  Port=1  Side=Left
  Vb1 : PMIOPort  Port=2  Side=Left
  Vc1 : PMIOPort  Port=3  Side=Left
  Vf2 : Outport
  Vf1 : Outport  Port=2
  wires:
  Voltage Measurement/1 -> Vf2/1, Sum/2, Scope/1
  PID Controller1/1 -> Vf1/1, Sum1/2, Scope2/1
  Sum/1 -> Sum1/1, Scope1/1
  Sum1/1 -> PID Controller1/1
  In MC1/1 -> Sum2/2
  Sum2/1 -> Sum/1
  Constant/1 -> Sum2/1
  connections:
  Diode1/LConn1 -- Voltage Measurement/LConn2 -- Diode5/LConn1 -- Diode3/LConn1
  Diode/LConn1 -- Va1/RConn1 -- Diode1/RConn1
  Diode2/LConn1 -- Vb1/RConn1 -- Diode3/RConn1
  Diode4/LConn1 -- Vc1/RConn1 -- Diode5/RConn1
  Diode/RConn1 -- Voltage Measurement/LConn1 -- Diode4/RConn1 -- Diode2/RConn1

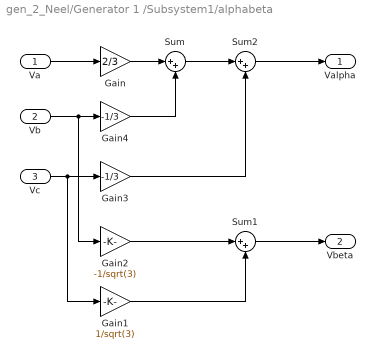
== system gen_2_Neel/Generator 1 /Subsystem1/alphabeta ==
  Va : Inport
  Vb : Inport  Port=2
  Vc : Inport  Port=3
  Gain : Gain  Gain=2/3
  Gain1 : Gain  Gain=1/sqrt(3)
  Gain2 : Gain  Gain=-1/sqrt(3)
  Gain3 : Gain  Gain=-1/3
  Gain4 : Gain  Gain=-1/3
  Sum : Sum  Inputs=|++
  Sum1 : Sum  Inputs=|++
  Sum2 : Sum  Inputs=|++
  Valpha : Outport
  Vbeta : Outport  Port=2
  wires:
  Vc/1 -> Gain1/1, Gain3/1
  Gain4/1 -> Sum/2
  Vb/1 -> Gain2/1, Gain4/1
  Sum1/1 -> Vbeta/1
  Sum/1 -> Sum2/1
  Gain/1 -> Sum/1
  Sum2/1 -> Valpha/1
  Va/1 -> Gain/1
  Gain2/1 -> Sum1/1
  Gain1/1 -> Sum1/2
  Gain3/1 -> Sum2/2

== system gen_2_Neel/Generator 1 /Subsystem1/dq ==
  theta : Inport
  Valpha : Inport  Port=2
  Vbeta : Inport  Port=3
  Fcn : Fcn  Expr=sin(u)
  Fcn1 : Fcn  Expr=cos(u)
  Product : Product
  Product1 : Product
  Sum1 : Sum  Inputs=|+-
  Vde : Outport
  wires:
  Vbeta/1 -> Product1/2
  theta/1 -> Fcn1/1, Fcn/1
  Fcn1/1 -> Product/1
  Valpha/1 -> Product/2
  Fcn/1 -> Product1/1
  Product1/1 -> Sum1/1
  Product/1 -> Sum1/2
  Sum1/1 -> Vde/1

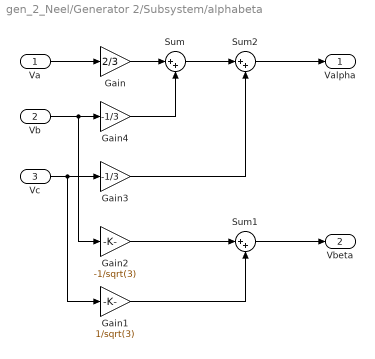
== system gen_2_Neel/Generator 2/Subsystem/alphabeta ==
  Va : Inport
  Vb : Inport  Port=2
  Vc : Inport  Port=3
  Gain : Gain  Gain=2/3
  Gain1 : Gain  Gain=1/sqrt(3)
  Gain2 : Gain  Gain=-1/sqrt(3)
  Gain3 : Gain  Gain=-1/3
  Gain4 : Gain  Gain=-1/3
  Sum : Sum  Inputs=|++
  Sum1 : Sum  Inputs=|++
  Sum2 : Sum  Inputs=|++
  Valpha : Outport
  Vbeta : Outport  Port=2
  wires:
  Vc/1 -> Gain1/1, Gain3/1
  Gain4/1 -> Sum/2
  Vb/1 -> Gain2/1, Gain4/1
  Sum1/1 -> Vbeta/1
  Sum/1 -> Sum2/1
  Gain/1 -> Sum/1
  Sum2/1 -> Valpha/1
  Va/1 -> Gain/1
  Gain2/1 -> Sum1/1
  Gain1/1 -> Sum1/2
  Gain3/1 -> Sum2/2

== system gen_2_Neel/Generator 2/Subsystem/dq ==
  theta : Inport
  Valpha : Inport  Port=2
  Vbeta : Inport  Port=3
  Fcn : Fcn  Expr=sin(u)
  Fcn1 : Fcn  Expr=cos(u)
  Product : Product
  Product1 : Product
  Sum1 : Sum  Inputs=|+-
  Vde : Outport
  wires:
  Vbeta/1 -> Product1/2
  theta/1 -> Fcn1/1, Fcn/1
  Fcn1/1 -> Product/1
  Valpha/1 -> Product/2
  Fcn/1 -> Product1/1
  Product1/1 -> Sum1/1
  Product/1 -> Sum1/2
  Sum1/1 -> Vde/1

== matlab function gen_2_Neel/MATLAB Function1 ==
  data: dc2 input; o2 output; o1 output; dc1 input; VMatch output
function [o2, o1,VMatch]= fcn(dc2,dc1)
persistent k1 k2 k3
if isempty(k1)
     k1= 0; 
end
if isempty(k2)
     k2= 0; 
end
if isempty(k3)
     k3= 0; 
end
o1=k1;
o2=k2;
VMatch=k3;
if dc1 < 387 && dc1>=389.6
    k1=0;
    k3 =0;
end 
if dc2 < 387 && dc2>=389.6 
    k2=0;
    k3 =0;
end
if dc1 > 387 && dc1 <=389.6 && dc2 > 387 && dc2 <=389.6
   k3=1;
end
end

== matlab function gen_2_Neel/MATLAB Function ==
  data: u input; y output; fMatch output
function [y,fMatch] = fcn(u)


persistent a 
if isempty(a)
     a= 0; 
end

persistent b 
if isempty(b)
     b= 0; 
end

% persistent t
% if isempty(t)
%      t= 0; 
% end

t=0.9;
b =37.7 - u;
fMatch=0;
if (u>37.3) && (u< 38.1)
    a=a;
elseif u<37.3 || u>38.1 
    a= b*t;
    fMatch=0;
end
if(u>36.8 && u<37.8)
    fMatch=1;
end
y=a;
end

== matlab function gen_2_Neel/MATLAB Function2 ==
  data: data1 input; u input; y output; data input
function y = fcn(data1, u, data)
persistent k
if isempty(k)
 k=0;
end
if ( u==0) 
    %if (diff(data1)>0)
    %    if (diff(data)>0)
        k=1;
    %    end
   % end
end
y=k;        
         
end

== matlab function gen_2_Neel/PhaseSync/MATLAB Function2 ==
  data: A1 input; u1 input; w2 output
function w2 = fcn(A1,u1)
w2=A1*sin(u1);
end

== matlab function gen_2_Neel/PhaseSync/MATLAB Function1 ==
  data: A input; u input; w1 output
function w1 = fcn(A,u)
w1=A*sin(u);
end
